simulink model "model1"  (R2021b)
settings: Solver=FixedStepAuto  StartTime=0.0  StopTime=10.0  FixedStep=0.001  RelTol=1e-3
undefined symbols (not defined in the file): DiscIntNeverNeededParam
libraries: simulink x2
settings Model: Creator=O  LastModifiedBy=wangzixuan

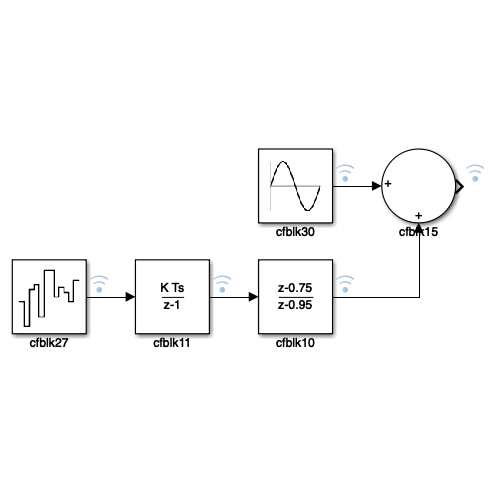
[thumbnail: Simulink's stored preview of the top-level diagram]
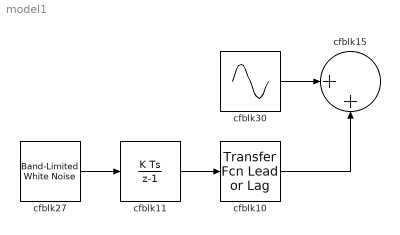
== system model1 ==
  cfblk10 : simulink/Discrete/Transfer Fcn Lead or Lag  PoleZ=0.95  ZeroZ=0.75  ICPrevOutput=0.0  ICPrevInput=0.0  DoSatur=off
      settings: SourceProductBaseCode=SL
  cfblk11 : DiscreteIntegrator  OutDataTypeStr=double  ICPrevOutput=DiscIntNeverNeededParam  ICPrevScaledInput=DiscIntNeverNeededParam
  cfblk15 : Sum  Inputs=|++  OutDataTypeStr=double
  cfblk27 : simulink/Sources/Band-Limited White Noise  Cov=[7496925313.772144]  Ts=0.1  seed=[9446467060.000000]
  cfblk30 : Sin  Amplitude=[-484213518.220894]  Bias=[-227187939.059104]  SampleTime=0
  wires:
  cfblk30/1 -> cfblk15/1
  cfblk11/1 -> cfblk10/1
  cfblk27/1 -> cfblk11/1
  cfblk10/1 -> cfblk15/2
